simulink model "magnetic_torquetofinish"  (R2020b)
settings: Solver=VariableStepAuto  StartTime=0.0  StopTime=10.0  RelTol=1e-3
libraries: vrlib x1
settings Model: Creator=jason  LastModifiedBy=jason

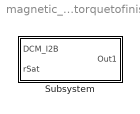
== system magnetic_torquetofinish ==
  Subsystem : Subsystem

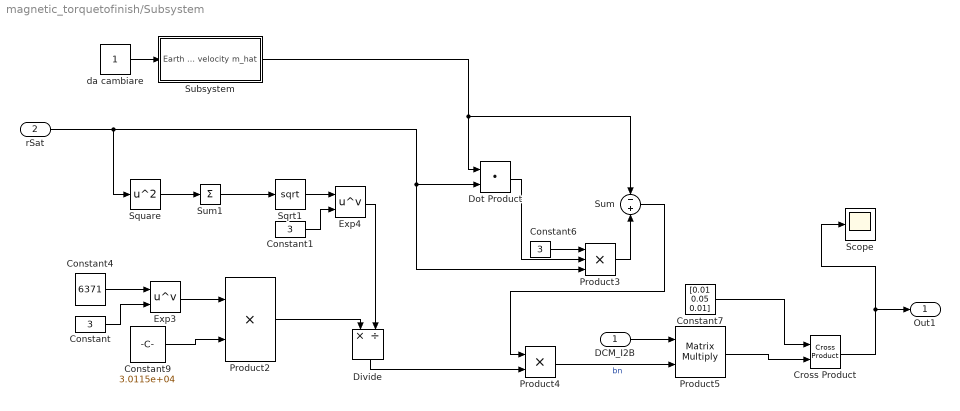
== system magnetic_torquetofinish/Subsystem ==
  DCM_I2B : Inport
  rSat : Inport  Port=2
  Constant : Constant  Value=3
  Constant1 : Constant  Value=3
  Constant4 : Constant  Value=6371
  Constant6 : Constant  Value=3
  Constant7 : Constant  Value=[0.01 0.05 0.01]
  Constant9 : Constant  Value=3.0115e+04
  Cross Product : vrlib/Utilities/Cross Product
  Divide : Product  Inputs=*/
  Dot Product : DotProduct  InputSameDT=on  OutDataTypeStr=Inherit: Inherit via internal rule
  Exp3 : Math  Operator=pow  SaturateOnIntegerOverflow=on
  Exp4 : Math  Operator=pow  SaturateOnIntegerOverflow=on
  Product2 : Product
  Product3 : Product  Inputs=3
  Product4 : Product
  Product5 : Product  Multiplication=Matrix(*)
  Scope : Scope
  Sqrt1 : Sqrt  SaturateOnIntegerOverflow=on
  Square : Math  Operator=square  SaturateOnIntegerOverflow=on
  Subsystem : Subsystem
  Sum : Sum  Inputs=-+
  Sum1 : Sum  Inputs=+
  da cambiare : Constant
  Out1 : Outport
  wires:
  Constant4/1 -> Exp3/1
  Product2/1 -> Divide/1
  Divide/1 -> Product4/2
  Constant6/1 -> Product3/1
  Dot Product/1 -> Product3/2
  Product3/1 -> Sum/2
  Sum/1 -> Product4/1
  Product4/1 -> Product5/2  "bn"
  Constant7/1 -> Cross Product/1
  Product5/1 -> Cross Product/2
  Cross Product/1 -> Scope/1, Out1/1
  Constant9/1 -> Product2/2
  Subsystem/1(m_hat) -> Sum/1, Dot Product/1
  Constant/1 -> Exp3/2
  Exp3/1 -> Product2/1
  Constant1/1 -> Exp4/2
  Exp4/1 -> Divide/2
  rSat/1 -> Square/1, Product3/3, Dot Product/2
  DCM_I2B/1 -> Product5/1
  Square/1 -> Sum1/1
  Sum1/1 -> Sqrt1/1
  Sqrt1/1 -> Exp4/1
  da cambiare/1 -> Subsystem/1(Earth angular velocity)

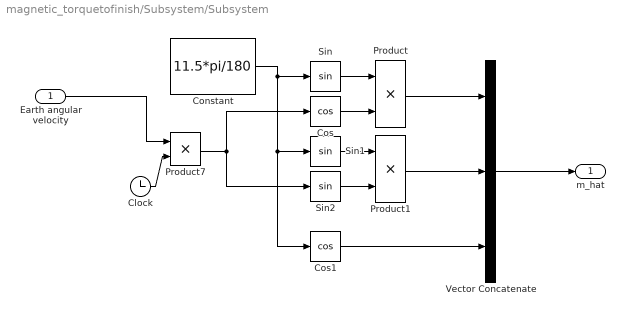
== system magnetic_torquetofinish/Subsystem/Subsystem ==
  Earth angular velocity : Inport
  Clock : Clock
  Constant : Constant  Value=11.5*pi/180
  Cos : Trigonometry  Operator=cos
  Cos1 : Trigonometry  Operator=cos
  Product : Product
  Product1 : Product
  Product7 : Product
  Sin : Trigonometry
  Sin1 : Trigonometry
  Sin2 : Trigonometry
  Vector Concatenate : Concatenate  NumInputs=3
  m_hat : Outport
  wires:
  Earth angular velocity/1 -> Product7/1
  Clock/1 -> Product7/2
  Sin1/1 -> Product1/1
  Sin/1 -> Product/1
  Product7/1 -> Cos/1, Sin2/1
  Product1/1 -> Vector Concatenate/2
  Product/1 -> Vector Concatenate/1
  Sin2/1 -> Product1/2
  Cos/1 -> Product/2
  Constant/1 -> Cos1/1, Sin1/1, Sin/1
  Cos1/1 -> Vector Concatenate/3
  Vector Concatenate/1 -> m_hat/1
